simulink model "Static_Compensator"  (R2021b)
settings: Solver=VariableStepAuto  StartTime=0.0  StopTime=30  RelTol=1e-3
undefined symbols (not defined in the file or in its folder): A, B, C, G_cl_DC, K
settings Model: Creator=Asus  LastModifiedBy=Asus

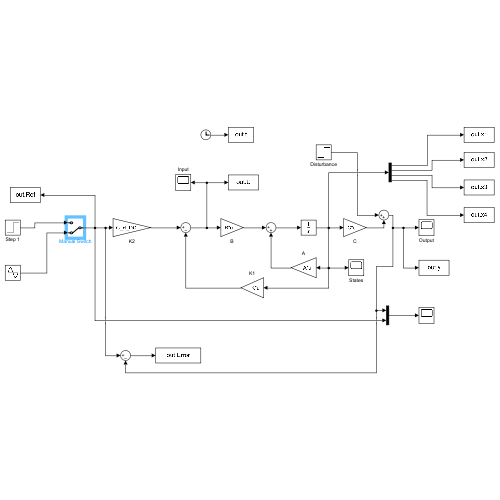
[thumbnail: Simulink's stored preview of the top-level diagram]
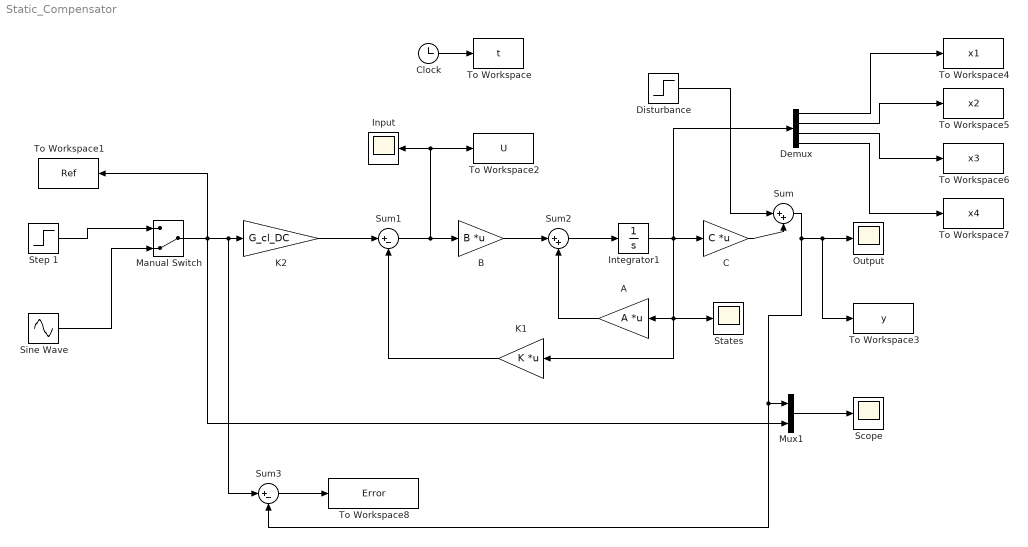
== system Static_Compensator ==
  A : Gain  Gain=A  Multiplication=Matrix(K*u)
  B : Gain  Gain=B  Multiplication=Matrix(K*u)
  C : Gain  Gain=C  Multiplication=Matrix(K*u)
  Clock : Clock
  Demux : Demux
  Disturbance : Step  Time=9  After=0  SampleTime=0
  Input : Scope
  Integrator1 : Integrator
  K1 : Gain  Gain=K  Multiplication=Matrix(K*u)
  K2 : Gain  Gain=G_cl_DC
  Manual Switch : ManualSwitch  CurrentSetting=0
  Mux1 : Mux  Inputs=2
  Output : Scope
  Scope : Scope
  Sine Wave : Sin  SampleTime=0
  States : Scope
  Step 1 : Step  After=10  SampleTime=0.001
  Sum : Sum  Inputs=|++
  Sum1 : Sum  Inputs=|+-
  Sum2 : Sum  Inputs=|++
  Sum3 : Sum  Inputs=|+-
  To Workspace : ToWorkspace  VariableName=t  SaveFormat=Timeseries  SampleTime=-1
  To Workspace1 : ToWorkspace  VariableName=Ref  SaveFormat=Timeseries  SampleTime=-1
  To Workspace2 : ToWorkspace  VariableName=U  SaveFormat=Timeseries  SampleTime=-1
  To Workspace3 : ToWorkspace  VariableName=y  SaveFormat=Timeseries  SampleTime=-1
  To Workspace4 : ToWorkspace  VariableName=x1  SaveFormat=Timeseries  SampleTime=-1
  To Workspace5 : ToWorkspace  VariableName=x2  SaveFormat=Timeseries  SampleTime=-1
  To Workspace6 : ToWorkspace  VariableName=x3  SaveFormat=Timeseries  SampleTime=-1
  To Workspace7 : ToWorkspace  VariableName=x4  SaveFormat=Timeseries  SampleTime=-1
  To Workspace8 : ToWorkspace  VariableName=Error  SaveFormat=Timeseries  SampleTime=-1
  wires:
  Integrator1/1 -> Demux/1, K1/1, States/1, A/1, C/1
  Demux/3 -> To Workspace6/1
  Demux/4 -> To Workspace7/1
  Demux/2 -> To Workspace5/1
  Sum2/1 -> Integrator1/1
  Sum1/1 -> Input/1, To Workspace2/1, B/1
  A/1 -> Sum2/2
  Mux1/1 -> Scope/1
  Clock/1 -> To Workspace/1
  C/1 -> Sum/2
  B/1 -> Sum2/1
  Demux/1 -> To Workspace4/1
  K1/1 -> Sum1/2
  K2/1 -> Sum1/1
  Sum/1 -> Sum3/2, Mux1/1, To Workspace3/1, Output/1
  Disturbance/1 -> Sum/1
  Manual Switch/1 -> To Workspace1/1, Mux1/2, Sum3/1, K2/1
  Step 1/1 -> Manual Switch/1
  Sine Wave/1 -> Manual Switch/2
  Sum3/1 -> To Workspace8/1
